simulink model "chap1_1"  (Simulink 3.00)
settings: Solver=ode45  StartTime=0.0  StopTime=10  RelTol=1e-3

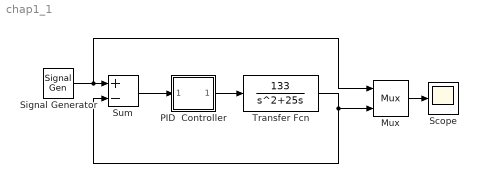
== system chap1_1 ==
  Mux : Mux  Inputs=2
      settings: DisplayOption=none
  PID  Controller : Subsystem  mask(PID Controller){@1=60, @2=1, @3=3}
      mask prompts: @1 "Proportional:"; @2 "Integral"; @3 "Derivative:"
      mask help:
      | Enter expressions for proportional, integral, and derivative terms.
      | P+I/s+Ds
      mask init:
      | P=@1; I=@2; D=@3;
      mask Help: This block implements a PID controller where parameters are entered for the Proportional, Integral and Derivative terms. Unmask this block to see how it works. The derivative term is implemented using a true derivative block.
      mask Display: disp('PID')
  Scope : Scope
      settings: TimeRange=10  YMin=-1  YMax=1  SaveToWorkspace=off  SaveName=ScopeData
  Signal Generator : SignalGenerator  WaveForm=sine  Amplitude=1  Frequency=0.2  Units=Hertz
  Sum : Sum  Inputs=+-  SaturateOnIntegerOverflow=on
  Transfer Fcn : TransferFcn  Numerator=[133]  Denominator=[1 25 0]
  wires:
  Mux/1 -> Scope/1
  Signal Generator/1 -> Sum/1, Mux/1
  Sum/1 -> PID  Controller/1(In_1)
  Transfer Fcn/1 -> Mux/2, Sum/2
  PID  Controller/1(Out_1) -> Transfer Fcn/1

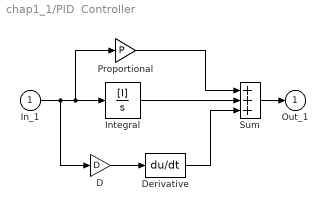
== system chap1_1/PID  Controller ==
  In_1 : Inport  Port=1  PortWidth=-1  SampleTime=-1  DataType=auto
      settings: SignalType=auto
  D : Gain  Gain=D  SaturateOnIntegerOverflow=on
  Derivative : Derivative
  Integral : TransferFcn  Numerator=[I]  Denominator=[1 0]
  Proportional : Gain  Gain=P  SaturateOnIntegerOverflow=on
  Sum : Sum  Inputs=+++  SaturateOnIntegerOverflow=on
  Out_1 : Outport  Port=1  InitialOutput=0
  wires:
  D/1 -> Derivative/1
  Sum/1 -> Out_1/1
  In_1/1 -> D/1, Proportional/1, Integral/1
  Derivative/1 -> Sum/3
  Integral/1 -> Sum/2
  Proportional/1 -> Sum/1
